simulink model "ActualDroneSetup"  (R2025a)
settings: Solver=VariableStepAuto  StartTime=0.0  StopTime=10.0  RelTol=1e-3
libraries: arduinosensorlib x1
settings Model: Creator=tobia  LastModifiedBy=tobia

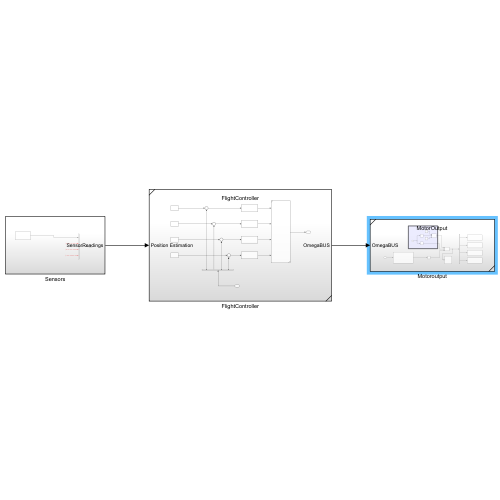
[thumbnail: Simulink's stored preview of the top-level diagram]
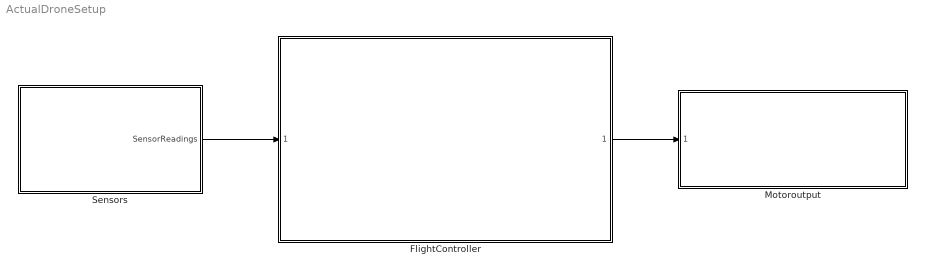
== system ActualDroneSetup ==
  FlightController : Subsystem  ReferencedSubsystem=FlightController
  Motoroutput : Subsystem  ReferencedSubsystem=MotorOutput
  Sensors : Subsystem
  wires:
  Sensors/1(SensorReadings) -> FlightController/1
  FlightController/1 -> Motoroutput/1

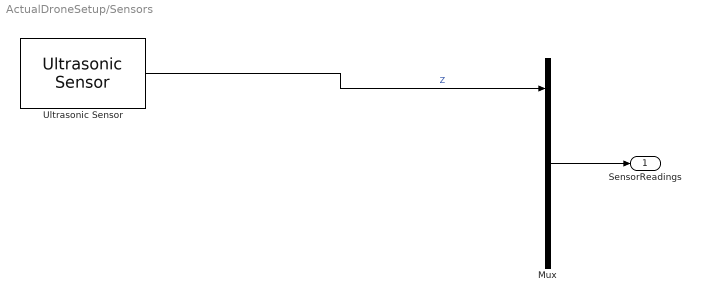
== system ActualDroneSetup/Sensors ==
  Mux : Mux
  Ultrasonic Sensor : arduinosensorlib/Ultrasonic Sensor  NumSignalPins=1  TrigPin=4  EchoPin=5  SignalPin=3  SampleTime_=0.1  blockPlatform=ARDUINO
  SensorReadings : Outport
  wires:
  Mux/1 -> SensorReadings/1
  Ultrasonic Sensor/1 -> Mux/1  "Z"
  ? -> Mux/2  "phi"
  ? -> Mux/3  "theta"
  ? -> Mux/4  "psi"
